simulink model "Exp3_Model"  (R2023b)
settings: Solver=ode3  StartTime=0.0  StopTime=time(end)  FixedStep=0.001  RelTol=1e-3
undefined symbols (not defined in the file): den, g, i_G, J, k_M, LT1D_FRICTION, m_G, num, r_P
settings Model: Creator=tunkarlu  LastModifiedBy=tunkarlu

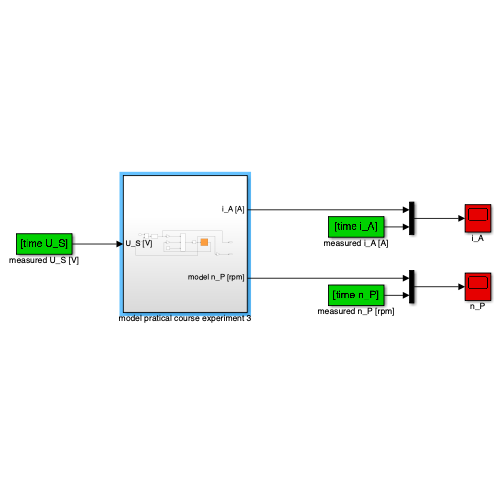
[thumbnail: Simulink's stored preview of the top-level diagram]
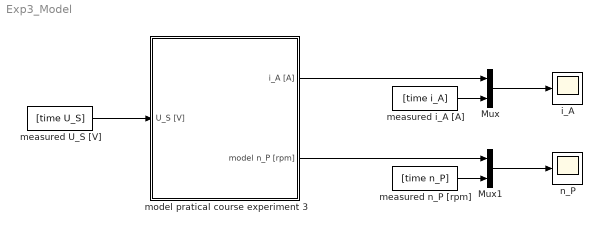
== system Exp3_Model ==
  Mux : Mux  Inputs=2
  Mux1 : Mux  Inputs=2
  i_A : Scope
  measured U_S [V] : FromWorkspace  VariableName=[time U_S]
  measured i_A [A] : FromWorkspace  VariableName=[time i_A]
  measured n_P [rpm] : FromWorkspace  VariableName=[time n_P]
  model pratical course experiment 3 : Subsystem
  n_P : Scope
  wires:
  Mux/1 -> i_A/1
  Mux1/1 -> n_P/1
  measured i_A [A]/1 -> Mux/2
  model pratical course experiment 3/1(i_A [A]) -> Mux/1
  model pratical course experiment 3/2(model n_P [rpm]) -> Mux1/1
  measured U_S [V]/1 -> model pratical course experiment 3/1(U_S [V])
  measured n_P [rpm]/1 -> Mux1/2

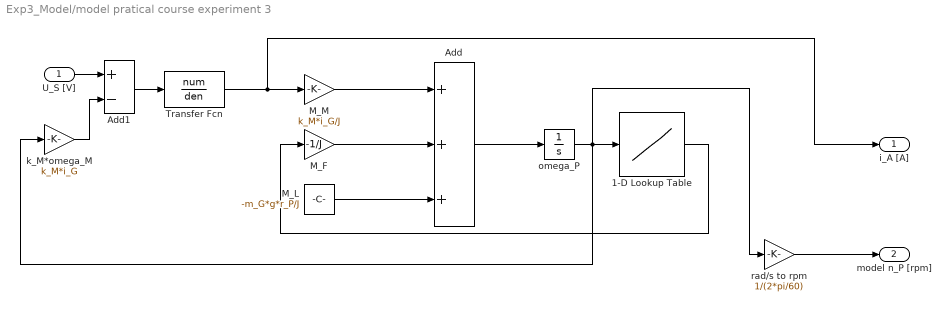
== system Exp3_Model/model pratical course experiment 3 ==
  U_S [V] : Inport
  1-D Lookup Table : Lookup_n-D  NumberOfTableDimensions=1  BreakpointsForDimension1=LT1D_FRICTION(1,:)  Table=LT1D_FRICTION(2,:)  InternalRulePriority=Speed  RndMeth=Simplest
  Add : Sum  Inputs=+++
  Add1 : Sum  Inputs=+-
  M_F : Gain  Gain=-1/J
  M_L : Constant  Value=-m_G*g*r_P/J
  M_M : Gain  Gain=k_M*i_G/J
  Transfer Fcn : TransferFcn  Numerator=num  Denominator=den
  k_M*omega_M : Gain  Gain=k_M*i_G
  omega_P : Integrator
  rad/s to rpm : Gain  Gain=1/(2*pi/60)
  i_A [A] : Outport
  model n_P [rpm] : Outport  Port=2
  wires:
  rad/s to rpm/1 -> model n_P [rpm]/1
  1-D Lookup Table/1 -> M_F/1
  M_L/1 -> Add/3
  Add/1 -> omega_P/1
  M_M/1 -> Add/1
  Transfer Fcn/1 -> i_A [A]/1, M_M/1
  omega_P/1 -> k_M*omega_M/1, 1-D Lookup Table/1, rad/s to rpm/1
  M_F/1 -> Add/2
  U_S [V]/1 -> Add1/1
  Add1/1 -> Transfer Fcn/1
  k_M*omega_M/1 -> Add1/2
